simulink model "ControllerStateModel_Harness1_replacement"  (R2024b)
settings: Solver=FixedStepAuto  StartTime=0.0  StopTime=10.0  FixedStep=0.01  RelTol=1e-3
undefined symbols (not defined in the file or in its folder): ALT_THRESHOLD, CLIMB_PITCH_CMD, Controller, GAIN, PERSISTENCT, STALL_SPEED
libraries: sldvlib x7, simulink x5
settings Model: DataDictionary=ControllerModel.sldd  DVDesignModelName=ControllerStateModel_Harness1  Creator=MBD_PRO  LastModifiedBy=MBD_PRO
settings ConfigComp: DVMode=PropertyProving  DVTestSuiteOptimization=Auto  DVDefectChecker=on  DVDetectOutOfBounds=on  DVModelReferenceHarness=on  DVHarnessSource=Signal Editor

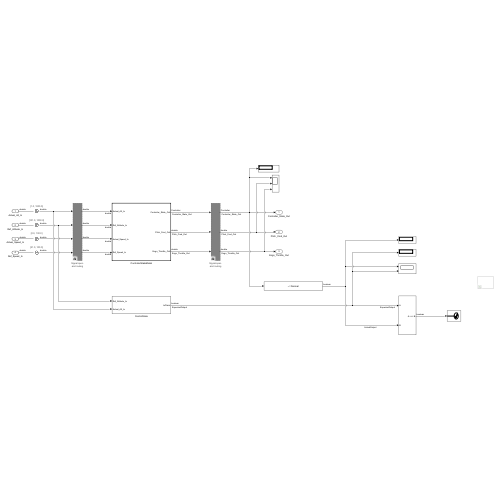
[thumbnail: Simulink's stored preview of the top-level diagram]
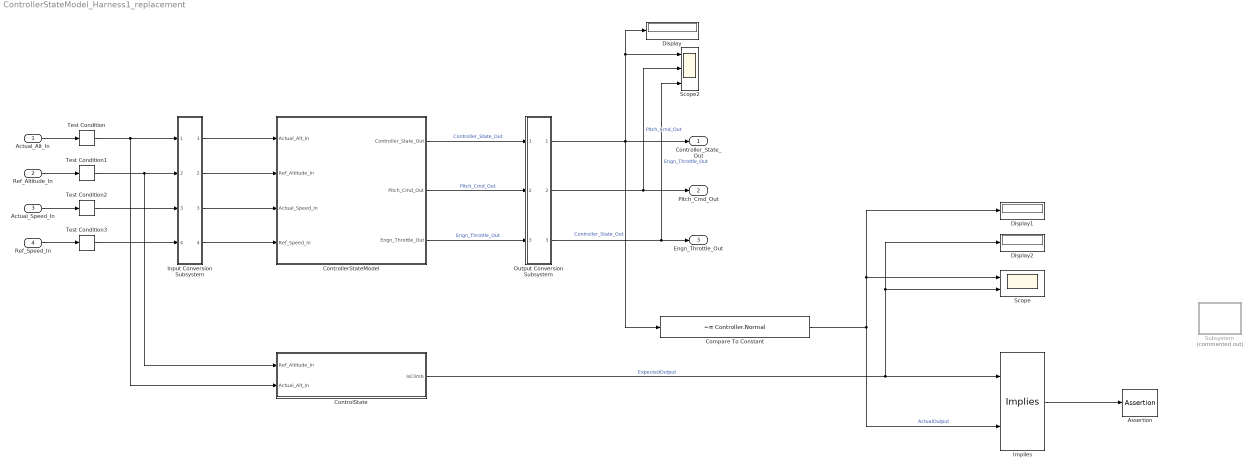
== system ControllerStateModel_Harness1_replacement ==
  Actual_Alt_In : Inport
  Ref_Altitude_In : Inport  Port=2
  Actual_Speed_In : Inport  Port=3
  Ref_Speed_In : Inport  Port=4
  Assertion : Assertion
  Compare To Constant : simulink/Logic and Bit Operations/Compare To Constant  relop=~=  const=Controller.Normal  OutDataTypeStr=boolean
  ControlState : Subsystem
  ControllerStateModel : Subsystem  TreatAsAtomicUnit=on  mask(Sldv ModelReference(Model name:ControllerStateModel) Replacement){ModelName=ControllerStateModel, ParameterArgumentNames=[], ParameterArgumentValuesAsString=, SimulationMode=Normal}
      mask help: Replacement for the Model Reference block that references the model ControllerStateModel. If Model arguments are specified on the Model Reference block, then they will appear in the mask parameters.
  Display : Display
  Display1 : Display
  Display2 : Display
  Implies : sldvlib/Verification Utilities/Implies
  Input Conversion Subsystem : Subsystem  Tag=__SLT_ICS__  Description=|
      | Signal spec.
      | and routing
      settings: AttributesFormatString=%<Description>
  Output Conversion Subsystem : Subsystem  Tag=__SLT_OCS__  Description=|
      | Signal spec.
      | and routing
      settings: AttributesFormatString=%<Description>
  Scope : Scope  NumInputPorts=2
  Scope2 : Scope  NumInputPorts=3
  Subsystem : Subsystem  Commented=on
  Test Condition : sldvlib/Objectives and Constraints/Test Condition  enabled=on  customAVTBlockType=Test Condition  intervals=[1.0, 1000.0]  initial=off  dispValues=on  outEnabled=on
      settings: AttributesFormatString=%<intervals>
  Test Condition1 : sldvlib/Objectives and Constraints/Test Condition  enabled=on  customAVTBlockType=Test Condition  intervals=[101.0, 1000.0]  initial=off  dispValues=on  outEnabled=on
      settings: AttributesFormatString=%<intervals>
  Test Condition2 : sldvlib/Objectives and Constraints/Test Condition  enabled=on  customAVTBlockType=Test Condition  intervals=[0.0, 100.0]  initial=off  dispValues=on  outEnabled=on
      settings: AttributesFormatString=%<intervals>
  Test Condition3 : sldvlib/Objectives and Constraints/Test Condition  enabled=on  customAVTBlockType=Test Condition  intervals=[21.0, 100.0]  initial=off  dispValues=on  outEnabled=on
      settings: AttributesFormatString=%<intervals>
  Controller_State_Out : Outport
  Pitch_Cmd_Out : Outport  Port=2
  Engn_Throttle_Out : Outport  Port=3
  wires:
  Actual_Alt_In/1 -> Test Condition/1
  Ref_Altitude_In/1 -> Test Condition1/1
  Actual_Speed_In/1 -> Test Condition2/1
  Ref_Speed_In/1 -> Test Condition3/1
  Input Conversion Subsystem/1(Outport_1) -> ControllerStateModel/1(Actual_Alt_In)
  Input Conversion Subsystem/2(Outport_2) -> ControllerStateModel/2(Ref_Altitude_In)
  Input Conversion Subsystem/3(Outport_3) -> ControllerStateModel/3(Actual_Speed_In)
  Input Conversion Subsystem/4(Outport_4) -> ControllerStateModel/4(Ref_Speed_In)
  Output Conversion Subsystem/1(Outport_1) -> Controller_State_Out/1, Compare To Constant/1, Display/1, Scope2/1  "Controller_State_Out"
  Output Conversion Subsystem/3(Outport_3) -> Scope2/3, Engn_Throttle_Out/1  "Engn_Throttle_Out"
  Output Conversion Subsystem/2(Outport_2) -> Scope2/2, Pitch_Cmd_Out/1  "Pitch_Cmd_Out"
  Test Condition/1 -> ControlState/2(Actual_Alt_In), Input Conversion Subsystem/1(Inport_1)
  Test Condition1/1 -> Input Conversion Subsystem/2(Inport_2), ControlState/1(Ref_Altitude_In)
  Test Condition2/1 -> Input Conversion Subsystem/3(Inport_3)
  Test Condition3/1 -> Input Conversion Subsystem/4(Inport_4)
  ControlState/1(IsClimb) -> Scope/2, Display2/1, Implies/1  "ExpectedOutput"
  Implies/1 -> Assertion/1
  Compare To Constant/1 -> Implies/2, Scope/1, Display1/1  "ActualOutput"
  ControllerStateModel/1(Controller_State_Out) -> Output Conversion Subsystem/1(Inport_1)  "Controller_State_Out"
  ControllerStateModel/2(Pitch_Cmd_Out) -> Output Conversion Subsystem/2(Inport_2)  "Pitch_Cmd_Out"
  ControllerStateModel/3(Engn_Throttle_Out) -> Output Conversion Subsystem/3(Inport_3)  "Engn_Throttle_Out"

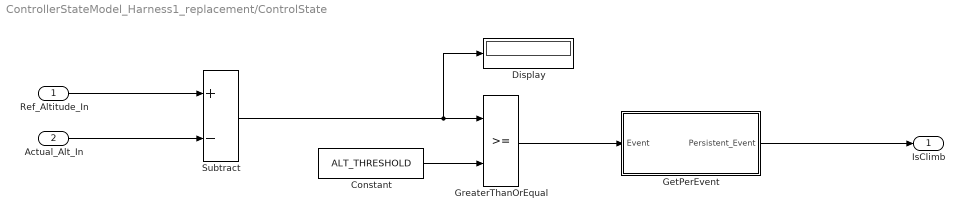
== system ControllerStateModel_Harness1_replacement/ControlState ==
  Ref_Altitude_In : Inport
  Actual_Alt_In : Inport  Port=2
  Constant : Constant  Value=ALT_THRESHOLD
  Display : Display
  GetPerEvent : Subsystem
  GreaterThanOrEqual : RelationalOperator  OutDataTypeStr=boolean  RndMeth=Simplest  InputSameDT=off
  Subtract : Sum  Inputs=+-
  IsClimb : Outport
  wires:
  Constant/1 -> GreaterThanOrEqual/2
  GreaterThanOrEqual/1 -> GetPerEvent/1(Event)
  Subtract/1 -> Display/1, GreaterThanOrEqual/1
  Ref_Altitude_In/1 -> Subtract/1
  Actual_Alt_In/1 -> Subtract/2
  GetPerEvent/1(Persistent_Event) -> IsClimb/1

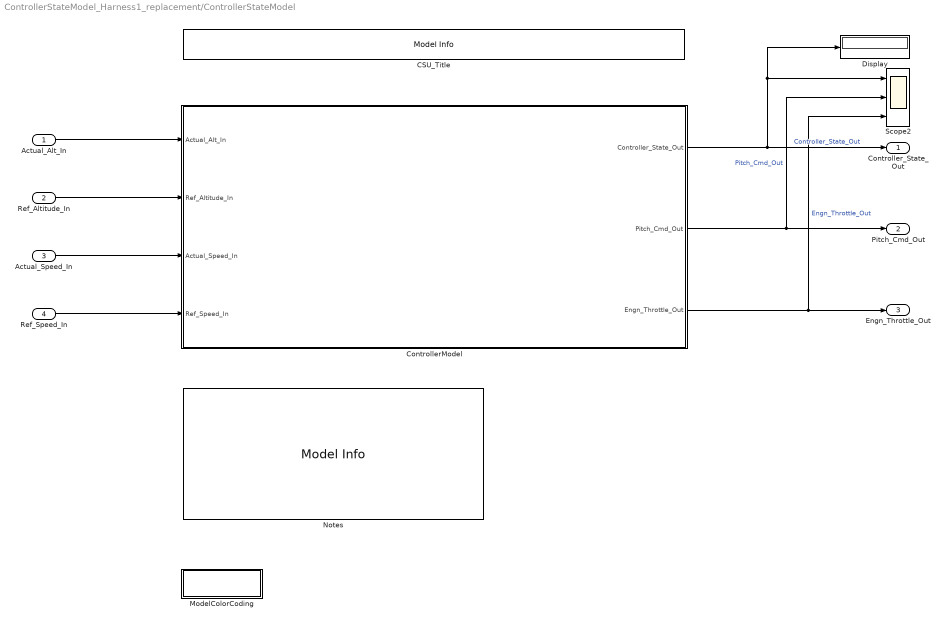
== system ControllerStateModel_Harness1_replacement/ControllerStateModel ==
  Actual_Alt_In : Inport  OutDataTypeStr=double  PortDimensions=1  SampleTime=[0.01,0]
  Ref_Altitude_In : Inport  Port=2  OutDataTypeStr=double  PortDimensions=1  SampleTime=[0.01,0]
  Actual_Speed_In : Inport  Port=3  OutDataTypeStr=double  PortDimensions=1  SampleTime=[0.01,0]
  Ref_Speed_In : Inport  Port=4  OutDataTypeStr=double  PortDimensions=1  SampleTime=[0.01,0]
  CSU_Title : simulink/Model-Wide Utilities/Model Info  Frame=on  DisplayStringWithTags=CSU Title: %<ModelName>  HorizontalTextAlignment=Center  LeftAlignmentValue=0.5
  ControllerModel : Subsystem
  Display : Display
  ModelColorCoding : Subsystem
      mask Display: disp("Model Color Coding");
  Notes : simulink/Model-Wide Utilities/Model Info  Frame=on  DisplayStringWithTags=|  HorizontalTextAlignment=Left  LeftAlignmentValue=0.02
      | Notes:
      | 
      | A. Remarks:
      |     None
      | 
      | B. Model details
      |     CSU Name: ModelName: %<ModelName>
      |     Author: Author Name
      |     LastModifiedBy: Author Name
      |     Version and Instance: %<ModelVersion>
      |     LastModificationDate: %<LastModificationDate>
  Scope2 : Scope  NumInputPorts=3
  Controller_State_Out : Outport  OutDataTypeStr=Enum: Controller  PortDimensions=1  SampleTime=[0.01,0]
  Pitch_Cmd_Out : Outport  Port=2  OutDataTypeStr=double  PortDimensions=1  SampleTime=[0.01,0]
  Engn_Throttle_Out : Outport  Port=3  OutDataTypeStr=double  PortDimensions=1  SampleTime=[0.01,0]
  wires:
  ControllerModel/2(Pitch_Cmd_Out) -> Scope2/2, Pitch_Cmd_Out/1  "Pitch_Cmd_Out"
  ControllerModel/3(Engn_Throttle_Out) -> Scope2/3, Engn_Throttle_Out/1  "Engn_Throttle_Out"
  ControllerModel/1(Controller_State_Out) -> Display/1, Scope2/1, Controller_State_Out/1  "Controller_State_Out"
  Ref_Altitude_In/1 -> ControllerModel/2(Ref_Altitude_In)
  Ref_Speed_In/1 -> ControllerModel/4(Ref_Speed_In)
  Actual_Alt_In/1 -> ControllerModel/1(Actual_Alt_In)
  Actual_Speed_In/1 -> ControllerModel/3(Actual_Speed_In)

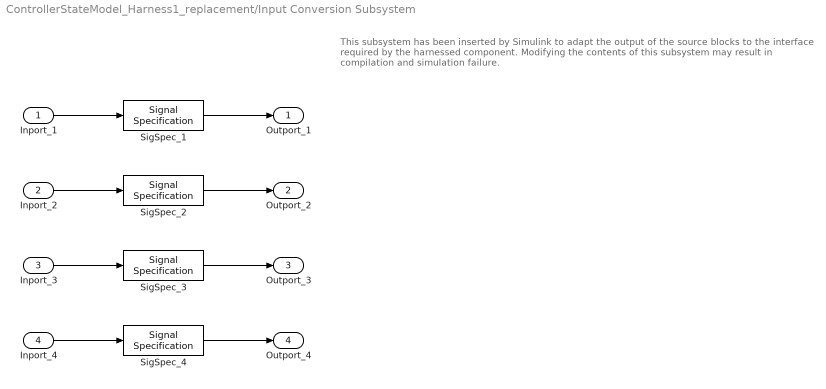
== system ControllerStateModel_Harness1_replacement/Input Conversion Subsystem ==
  note: This subsystem has been inserted by Simulink to adapt the output of the source blocks to the interface required by the harnessed component.
      |  Modifying the contents of this subsystem may result in compilation and simulation failure.
  Inport_1 : Inport
  Inport_2 : Inport  Port=2
  Inport_3 : Inport  Port=3
  Inport_4 : Inport  Port=4
  SigSpec_{1..4} (4 alike) : SignalSpecification  OutDataTypeStr=double  Dimensions=[1]  SampleTime=0.01
  Outport_1 : Outport
  Outport_2 : Outport  Port=2
  Outport_3 : Outport  Port=3
  Outport_4 : Outport  Port=4
  wires:
  SigSpec_1/1 -> Outport_1/1
  Inport_1/1 -> SigSpec_1/1
  SigSpec_2/1 -> Outport_2/1
  Inport_2/1 -> SigSpec_2/1
  SigSpec_3/1 -> Outport_3/1
  Inport_3/1 -> SigSpec_3/1
  SigSpec_4/1 -> Outport_4/1
  Inport_4/1 -> SigSpec_4/1

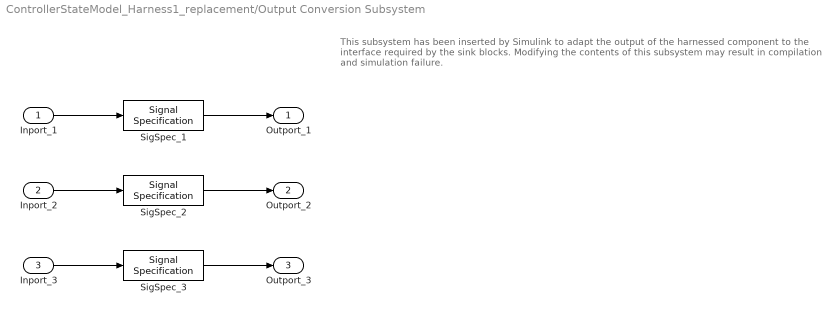
== system ControllerStateModel_Harness1_replacement/Output Conversion Subsystem ==
  note: This subsystem has been inserted by Simulink to adapt the output of the harnessed component to the interface required by the sink blocks.
      |  Modifying the contents of this subsystem may result in compilation and simulation failure.
  Inport_1 : Inport
  Inport_2 : Inport  Port=2
  Inport_3 : Inport  Port=3
  SigSpec_1 : SignalSpecification  OutDataTypeStr=Enum: Controller  Dimensions=[1]  SampleTime=0.01
  SigSpec_2 : SignalSpecification  OutDataTypeStr=double  Dimensions=[1]  SampleTime=0.01
  SigSpec_3 : SignalSpecification  OutDataTypeStr=double  Dimensions=[1]  SampleTime=0.01
  Outport_1 : Outport
  Outport_2 : Outport  Port=2
  Outport_3 : Outport  Port=3
  wires:
  Inport_1/1 -> SigSpec_1/1
  SigSpec_1/1 -> Outport_1/1
  Inport_2/1 -> SigSpec_2/1
  SigSpec_2/1 -> Outport_2/1
  Inport_3/1 -> SigSpec_3/1
  SigSpec_3/1 -> Outport_3/1

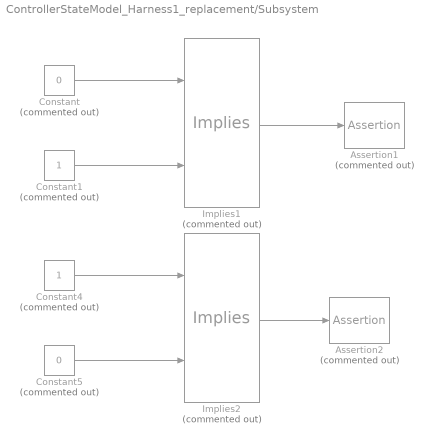
== system ControllerStateModel_Harness1_replacement/Subsystem ==
  Assertion1 : Assertion  Commented=on
  Assertion2 : Assertion  Commented=on
  Constant : Constant  Commented=on  Value=0  OutDataTypeStr=boolean
  Constant1 : Constant  Commented=on  OutDataTypeStr=boolean
  Constant4 : Constant  Commented=on  OutDataTypeStr=boolean
  Constant5 : Constant  Commented=on  Value=0  OutDataTypeStr=boolean
  Implies1 : sldvlib/Verification Utilities/Implies  Commented=on
  Implies2 : sldvlib/Verification Utilities/Implies  Commented=on
  wires:
  Constant1/1 -> Implies1/2
  Implies1/1 -> Assertion1/1
  Constant4/1 -> Implies2/1
  Implies2/1 -> Assertion2/1
  Constant/1 -> Implies1/1
  Constant5/1 -> Implies2/2

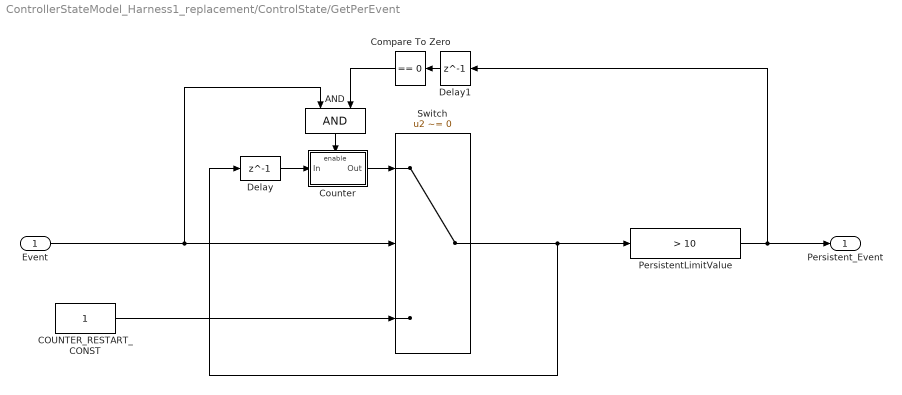
== system ControllerStateModel_Harness1_replacement/ControlState/GetPerEvent ==
  Event : Inport  OutDataTypeStr=boolean
  AND : Logic  AllPortsSameDT=off  OutDataTypeStr=boolean
  COUNTER_RESTART_CONST : Constant  OutDataTypeStr=uint32
  Compare To Zero : simulink/Logic and Bit Operations/Compare To Zero  relop===  OutDataTypeStr=boolean
  Counter : Subsystem  TreatAsAtomicUnit=on
  Delay : Delay  DelayLength=1  InitialCondition=0
  Delay1 : Delay  DelayLength=1  InitialCondition=0
  PersistentLimitValue : simulink/Logic and Bit Operations/Compare To Constant  relop=>  const=10  OutDataTypeStr=boolean
  Switch : Switch  Criteria=u2 ~= 0  SaturateOnIntegerOverflow=off  InputSameDT=off
  Persistent_Event : Outport  OutDataTypeStr=boolean
  wires:
  Event/1 -> Switch/2, AND/1
  Delay1/1 -> Compare To Zero/1
  Counter/1(Out) -> Switch/1
  PersistentLimitValue/1 -> Persistent_Event/1, Delay1/1
  Compare To Zero/1 -> AND/2
  Delay/1 -> Counter/1(In)
  Switch/1 -> Delay/1, PersistentLimitValue/1
  COUNTER_RESTART_CONST/1 -> Switch/3
  AND/1 -> Counter/Enable

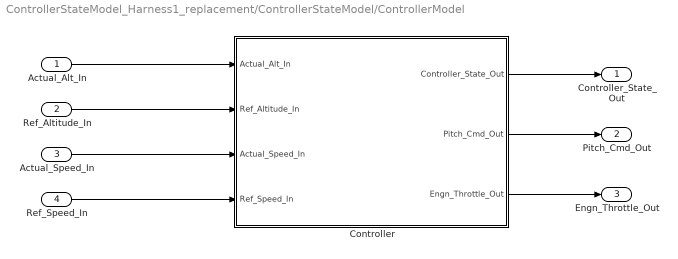
== system ControllerStateModel_Harness1_replacement/ControllerStateModel/ControllerModel ==
  Actual_Alt_In : Inport
  Ref_Altitude_In : Inport  Port=2
  Actual_Speed_In : Inport  Port=3
  Ref_Speed_In : Inport  Port=4
  Controller : Stateflow chart  TreatAsAtomicUnit=on
  Controller_State_Out : Outport
  Pitch_Cmd_Out : Outport  Port=2
  Engn_Throttle_Out : Outport  Port=3
  wires:
  Controller/1(Controller_State_Out) -> Controller_State_Out/1
  Ref_Speed_In/1 -> Controller/4(Ref_Speed_In)
  Actual_Speed_In/1 -> Controller/3(Actual_Speed_In)
  Actual_Alt_In/1 -> Controller/1(Actual_Alt_In)
  Ref_Altitude_In/1 -> Controller/2(Ref_Altitude_In)
  Controller/2(Pitch_Cmd_Out) -> Pitch_Cmd_Out/1
  Controller/3(Engn_Throttle_Out) -> Engn_Throttle_Out/1

== system ControllerStateModel_Harness1_replacement/ControllerStateModel/ModelColorCoding ==
  note: Model color coding
      |
      | Inport and Outport blocks color ( Cyan )
      | #00ffff
      |
      | Simulink Library blocks color (White)
      | #ffffff
      |
      | FCS ADE Library blocks color (Purple)
      | #00cc00
      |
      | Goto and From blocks color (Yellow)
      | #ffff00
      |
      | Disabled Link Library blocks color (Gray)
      | #ff7c7e
      |
      | Internal Subsystem color (Blue)
      | #55aaff
      |
      | Embeded matlab function (Gray)
      | #a6a6a6
      |
      | Outer Subsystem color (TBD)
      | #b746ff
      |
      | Model Reference block color (Orange)
      | #ff6929
      |
      | Any Remark or Note to the block color(TBD)
      | #aa0000

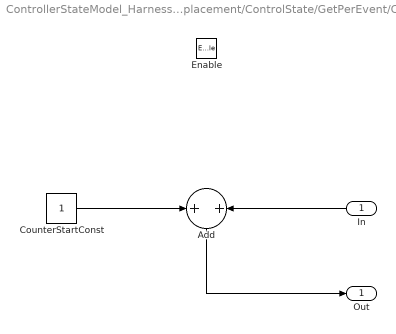
== system ControllerStateModel_Harness1_replacement/ControlState/GetPerEvent/Counter ==
  In : Inport
  Enable : EnablePort
  Add : Sum
  CounterStartConst : Constant  OutDataTypeStr=uint32
  Out : Outport
  wires:
  In/1 -> Add/2
  Add/1 -> Out/1
  CounterStartConst/1 -> Add/1

== stateflow chart ControllerStateModel_Harness1_replacement/ControllerStateModel/ControllerModel/Controller ==
  state Normal
    entry:
    Controller_State_Out = Controller.Normal;
    count_stall_recov = 1;
    count_climb = 1;
    during:
    %
    % Transition from state Normal to Climb
    if ((Ref_Altitude_In - Actual_Alt_In) >= ALT_THRESHOLD)
    if (count_climb >= PERSISTENCT)
    Controller_State_Out = Controller.Climb;
    else
    count_climb = count_climb + 1;
    end
    else
    count_climb = 1;
    end
    %
    % Transition from state Normal to StallRecovery
    if Actual_Speed_In < STALL_SPEED
    if (count_stall_recov >= PERSISTENCT)
    Controller_State_Out = Controller.StallRecovery;
    else
    count_stall_recov = count_stall_recov + 1;
    end
    else
    count_stall_recov = 1;
    end
    %
    % Computation
    Pitch_Cmd_Out = (Ref_Altitude_In - Actual_Alt_In) * GAIN;
    Engn_Throttle_Out = (Ref_Speed_In - Actual_Speed_In) * GAIN;
    exit:
  state Climb
    entry:
    Controller_State_Out = Controller.Climb
    count_stall_recov = 1;
    count_normal = 1;
    during:
    %
    % Transition from state Climb to Normal
    if Actual_Alt_In > Ref_Altitude_In
    if (count_normal >= PERSISTENCT)
    Controller_State_Out = Controller.Normal;
    else
    count_normal = count_normal + 1;
    end
    else
    count_normal = 1;
    end
    %
    % Transition from state Climb to StallRecovery
    if Actual_Speed_In < STALL_SPEED
    if (count_stall_recov >= PERSISTENCT)
    Controller_State_Out = Controller.StallRecovery;
    else
    count_stall_recov = count_stall_recov + 1;
    end
    else
    count_stall_recov = 1;
    end
    %
    % Computation
    Pitch_Cmd_Out = CLIMB_PITCH_CMD;
    Engn_Throttle_Out = 100.0;
    exit:
  state StallRecovery
    entry:
    Controller_State_Out = Controller.StallRecovery
    count_climb = 1;
    during:
    % Transition from state StallRecovery to Normal
    if Actual_Speed_In > STALL_SPEED
    if (count_climb >= PERSISTENCT)
    Controller_State_Out = Controller.Normal;
    else
    count_climb = count_climb + 1;
    end
    else
    count_climb = 1;
    end
    % Computation
    Pitch_Cmd_Out = 0.0;
    Engn_Throttle_Out = 100.0;
    exit:
  (default) -> Normal
  Climb -> Normal [order 2] : [Controller_State_Out == Controller.Normal]
  Normal -> Climb [order 2] : [Controller_State_Out == Controller.Climb]
  StallRecovery -> Normal : [Controller_State_Out == Controller.Normal]
  Normal -> StallRecovery [order 1] : [Controller_State_Out == Controller.StallRecovery]
  Climb -> StallRecovery [order 1] : [Controller_State_Out == Controller.StallRecovery]
  data: Actual_Alt_In input; Ref_Altitude_In input; Actual_Speed_In input; Ref_Speed_In input; PERSISTENCT parameter double; Controller_State_Out output; STALL_SPEED parameter; count_stall_recov local; count_climb local; count_normal local; Pitch_Cmd_Out output =0.0; Engn_Throttle_Out output =0.0; GAIN parameter; CLIMB_PITCH_CMD parameter; ALT_THRESHOLD parameter
